simulink model "ThreePhase_Energy"  (R2024b)
settings: Solver=FixedStepAuto  StartTime=0.0  StopTime=Tsim  FixedStep=1e-5  RelTol=1e-3
values from neighbouring files (symbols this model uses):
  C = 2e-3    (= 0.002)    [PR_init_run.m]    (also in PowerClarke.m = [1 1 1;1 -1 0; 1 0 -1;])
  eng_ki = 1000    [PR_init_run.m]
  eng_kp = 20    [PR_init_run.m]
  Eref1 = 3*(0.5)*C*Vdc^2    (= 1920)    [PR_init_run.m]
  Eref2 = 0    [PR_init_run.m]
  Eref3 = 0    [PR_init_run.m]
  f = 50    [PR_init_run.m]
  Ki = 120    [PR_init_run.m]
  ki = 1000    [PR_init_run.m]
  Kp = 1    [PR_init_run.m]
  kp = 20    [PR_init_run.m]
  L = 1.3e-3    (= 0.0013)    [PR_init_run.m]
  max_i = 30    [PR_init_run.m]
  P = 10e3    (= 10000)    [PR_init_run.m]
  Ptrf = [1 1 1;1 -1 0; 1 0 -1;]    [PR_init_run.m]
  Q = 0    [PR_init_run.m]    (also in SOGI_bode.m = 3)
  Q1ref = -15e3    (= -15000)    [PR_init_run.m]
  R = 1e-2    (= 0.01)    [PR_init_run.m]
  Rcap = 50e-3    (= 0.05)    [PR_init_run.m]
  sogi_ki = 30    [PR_init_run.m]
  sogi_kp = 0.5    [PR_init_run.m]
  Tdist = 0.3    [PR_init_run.m]
  TQ = 0.08    [PR_init_run.m]
  Tstep = 0.06    [PR_init_run.m]
  Vdc = 800    [PR_init_run.m]
  Vpeak = V2*sqrt(2)    [PR_init_run.m]
  w = 2*pi*f    (= 314.159265359)    [PR_init_run.m]    (also in SOGI_bode.m)
  wc = 0.6283    [PR_init_run.m]
libraries: spsControlledVoltageSourceLib x9, simulink x4, spsControlledCurrentSourceLib x3, spsCurrentMeasurementLib x3, spsSeriesRLCBranchLib x3, spsVoltageMeasurementLib x3, spsAlphaBetaZerotodq0Lib x2, spsThreePhaseVIMeasurementLib x2, spsGroundLib x1, spsThreePhaseSeriesRLCBranchLib x1, sps_lib x1
settings Model: Creator=sproj  LastModifiedBy=sproj

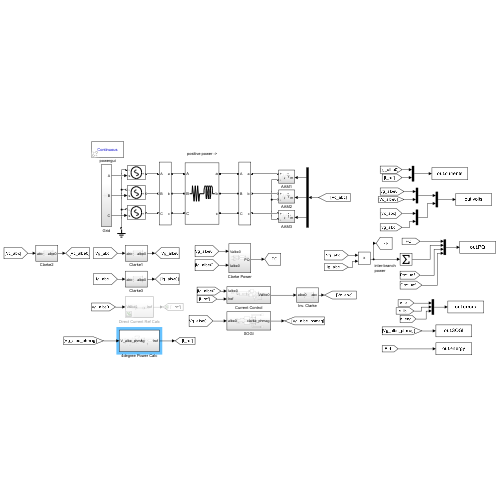
[thumbnail: Simulink's stored preview of the top-level diagram]
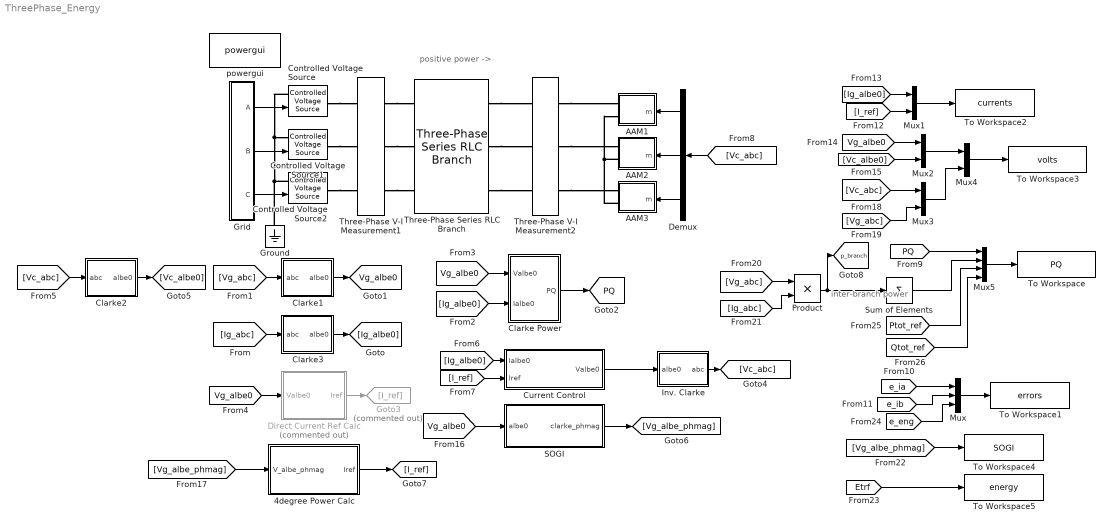
== system ThreePhase_Energy ==
  note: positive power ->
  note: inter-branch
      | power
  4degree Power Calc : Subsystem
  AAM1 : Subsystem
  AAM2 : Subsystem
  AAM3 : Subsystem
  Clarke Power : Subsystem
  Clarke1 : Subsystem
  Clarke2 : Subsystem
  Clarke3 : Subsystem
  Controlled Voltage Source : spsControlledVoltageSourceLib/Controlled Voltage Source  Initialize=on  Source_Type=AC  Amplitude=0  Phase=0  Frequency=0  Measurements=None
  Controlled Voltage Source1 : spsControlledVoltageSourceLib/Controlled Voltage Source  Initialize=on  Source_Type=AC  Amplitude=0  Phase=0  Frequency=0  Measurements=None
  Controlled Voltage Source2 : spsControlledVoltageSourceLib/Controlled Voltage Source  Initialize=on  Source_Type=AC  Amplitude=0  Phase=0  Frequency=0  Measurements=None
  Current Control : Subsystem
  Demux : Demux  Outputs=3
  Direct Current Ref Calc : Subsystem  Commented=on
  Goto3 : Goto  Commented=on  GotoTag=I_ref
  Grid : Subsystem
  Ground : spsGroundLib/Ground  LConnTagsString=a
  Inv. Clarke : Subsystem
  Mux : Mux  Inputs=3
  Mux{1..4} (4 alike) : Mux  Inputs=2
  Mux5 : Mux
  Product : Product
  SOGI : Subsystem
  Sum of Elements : Sum  Inputs=+
  Three-Phase Series RLC Branch : spsThreePhaseSeriesRLCBranchLib/Three-Phase Series RLC Branch  LConnTagsString=A|B|C  RConnTagsString=A|B|C  BranchType=RL  Resistance=R  Inductance=L  Capacitance=1e-6  Measurements=None
  Three-Phase V-I Measurement1 : spsThreePhaseVIMeasurementLib/Three-Phase V-I Measurement  VoltageMeasurement=phase-to-ground  SetLabelV=on  LabelV=Vg_abc  Vpu=off  VpuLL=off  CurrentMeasurement=yes  SetLabelI=on  LabelI=Ig_abc  Ipu=off  Pbase=100e6  Vbase=500e3  OutputType=Complex  PhasorSimulation=off  PSBequivalent=0
  Three-Phase V-I Measurement2 : spsThreePhaseVIMeasurementLib/Three-Phase V-I Measurement  VoltageMeasurement=phase-to-ground  SetLabelV=on  LabelV=Vc_abc  Vpu=off  VpuLL=off  CurrentMeasurement=yes  SetLabelI=on  LabelI=Ic_abc  Ipu=off  Pbase=100e6  Vbase=500e3  OutputType=Complex  PhasorSimulation=off  PSBequivalent=0
  To Workspace : ToWorkspace  VariableName=PQ  SaveFormat=Structure With Time  SampleTime=-1
  To Workspace1 : ToWorkspace  VariableName=errors  SaveFormat=Structure With Time  SampleTime=-1
  To Workspace2 : ToWorkspace  VariableName=currents  SaveFormat=Structure With Time  SampleTime=-1
  To Workspace3 : ToWorkspace  VariableName=volts  SaveFormat=Structure With Time  SampleTime=-1
  To Workspace4 : ToWorkspace  VariableName=SOGI  SaveFormat=Structure With Time  SampleTime=-1
  To Workspace5 : ToWorkspace  VariableName=energy  SaveFormat=Structure With Time  SampleTime=-1
  powergui : sps_lib/powergui  Priority=1  SimulationMode=Continuous  SampleTime=50e-6  frequency=60  Iterations=50  frequencyindice=0  Pbase=100e6  ErrMax=1e-4  UnitsV=kV  UnitsW=MW  buscounter=0  FunctionMessages=off  echomessages=off  EnableUseOfTLC=off  CurrentSourceSwitches=off  DisableSnubberDevices=off  DisableRonSwitches=off  DisableVfSwitches=off  DisplayEquations=off  AutomaticDiscreteSolvers=off  SolverType=Tustin/Backward Euler (TBE)  Interpol=off  ExternalGateDelay=off  methode=off  Ts=100  x0status=blocks  SPID=on  SwTol=0  HookPort=off  NonlinearTolerance=1e-4  nMaxIteration=100  ContinueOnMaxIteration=off  RestoreLinks=warning  ResistiveCurrentMeasurement=off  Frange=[0:2:500]  Ylog=off  Xlog=on  ShowGrid=off  save=off  variable=ZData  structure=0  ZoomFFT=off  StartTime=0.0  cycles=1  DisplayStyle=1  fundamental=60  FreqAxis=off  MaxFrequency=1000  frequencyindicesteady=1  RmsSteady=1  display=off
  tag scope: PQ=global, Vg_albe0=global, p_branch=global
  wires:
  Grid/2(B) -> Controlled Voltage Source1/1
  Grid/1(A) -> Controlled Voltage Source/1
  Grid/3(C) -> Controlled Voltage Source2/1
  [Ig_abc] -> Clarke3/1(abc)
  Clarke3/1(albe0) -> [Ig_albe0]
  [Vg_abc] -> Clarke1/1(abc)
  Clarke1/1(albe0) -> [Vg_albe0]
  [Ig_albe0] -> Clarke Power/2(Ialbe0)
  [Vg_albe0] -> Clarke Power/1(Valbe0)
  [Vg_albe0] -> Direct Current Ref Calc/1(Valbe0)
  Clarke Power/1(PQ) -> [PQ]
  [Ig_albe0] -> Current Control/1(Ialbe0)
  Direct Current Ref Calc/1(Iref) -> Goto3/1
  [I_ref] -> Current Control/2(Iref)
  Inv. Clarke/1(abc) -> [Vc_abc]
  [Vc_abc] -> Demux/1
  [e_ia] -> Mux/1
  [e_ib] -> Mux/2
  Mux/1 -> To Workspace1/1
  [Ig_albe0] -> Mux1/1
  [I_ref] -> Mux1/2
  Mux1/1 -> To Workspace2/1
  Current Control/1(Valbe0) -> Inv. Clarke/1(albe0)
  Demux/2 -> AAM2/1(m)
  Demux/1 -> AAM1/1(m)
  Demux/3 -> AAM3/1(m)
  [Vg_albe0] -> Mux2/1
  Clarke2/1(albe0) -> [Vc_albe0]
  [Vc_abc] -> Clarke2/1(abc)
  [Vc_albe0] -> Mux2/2
  [Vg_albe0] -> SOGI/1(albe0)
  SOGI/1(clarke_phmag) -> [Vg_albe_phmag]
  [Vg_albe_phmag] -> 4degree Power Calc/1(V_albe_phmag)
  [Vc_abc] -> Mux3/1
  [Vg_abc] -> Mux3/2
  Mux2/1 -> Mux4/1
  Mux3/1 -> Mux4/2
  Mux4/1 -> To Workspace3/1
  [Vg_abc] -> Product/1
  [Ig_abc] -> Product/2
  Product/1 -> Sum of Elements/1, [p_branch]
  [PQ] -> Mux5/1
  Sum of Elements/1 -> Mux5/2
  Mux5/1 -> To Workspace/1
  4degree Power Calc/1(Iref) -> [I_ref]
  [Vg_albe_phmag] -> To Workspace4/1
  [Etrf] -> To Workspace5/1
  [e_eng] -> Mux/3
  [Ptot_ref] -> Mux5/3
  [Qtot_ref] -> Mux5/4
  connections:
  Controlled Voltage Source1/LConn1 -- Controlled Voltage Source2/LConn1 -- Ground/LConn1 -- Controlled Voltage Source/LConn1
  Three-Phase Series RLC Branch/RConn1 -- Three-Phase V-I Measurement2/LConn1
  Three-Phase Series RLC Branch/RConn2 -- Three-Phase V-I Measurement2/LConn2
  Three-Phase Series RLC Branch/RConn3 -- Three-Phase V-I Measurement2/LConn3
  Three-Phase V-I Measurement2/RConn3 -- AAM3/RConn1
  Three-Phase V-I Measurement2/RConn2 -- AAM2/RConn1
  Three-Phase V-I Measurement2/RConn1 -- AAM1/RConn1
  Controlled Voltage Source/RConn1 -- Three-Phase V-I Measurement1/LConn1
  Controlled Voltage Source1/RConn1 -- Three-Phase V-I Measurement1/LConn2
  Controlled Voltage Source2/RConn1 -- Three-Phase V-I Measurement1/LConn3
  Three-Phase V-I Measurement1/RConn1 -- Three-Phase Series RLC Branch/LConn1
  Three-Phase V-I Measurement1/RConn2 -- Three-Phase Series RLC Branch/LConn2
  Three-Phase V-I Measurement1/RConn3 -- Three-Phase Series RLC Branch/LConn3
  AAM2/RConn2 -- AAM1/RConn2 -- AAM3/RConn2

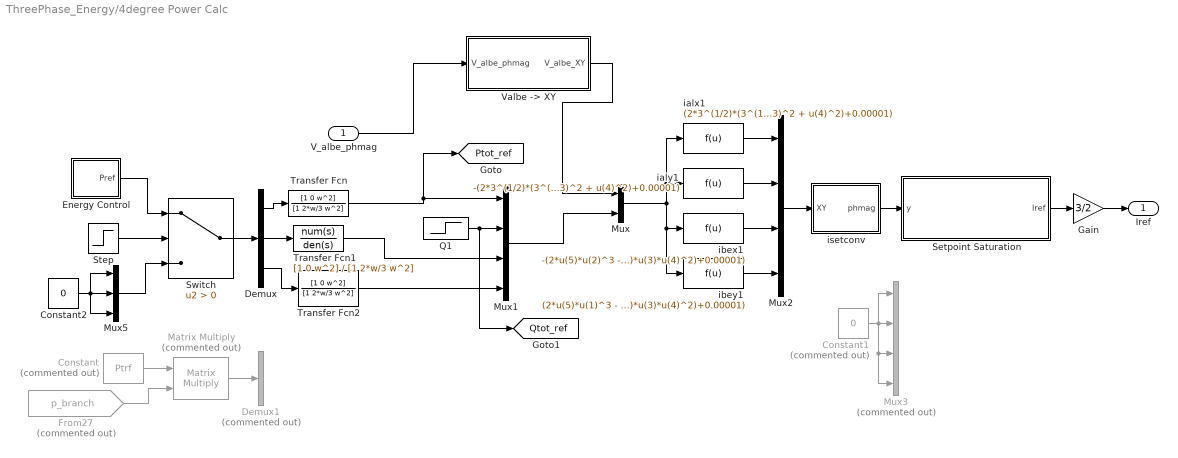
== system ThreePhase_Energy/4degree Power Calc ==
  V_albe_phmag : Inport
  Constant : Constant  Commented=on  Value=Ptrf
  Constant1 : Constant  Commented=on  Value=0
  Constant2 : Constant  Value=0
  Demux : Demux  Outputs=3
  Demux1 : Demux  Commented=on  Outputs=3
  Energy Control : Subsystem
  From27 : From  Commented=on  GotoTag=p_branch  TagVisibility=global
  Gain : Gain  Gain=3/2
  Matrix Multiply : Product  Commented=on  Multiplication=Matrix(*)
  Mux : Mux  Inputs=2
  Mux1 : Mux
  Mux2 : Mux
  Mux3 : Mux  Commented=on
  Mux5 : Mux  Inputs=3
  Q1 : Step  Time=TQ  After=Q1ref  SampleTime=0
  Setpoint Saturation : Subsystem
  Step : Step  Time=Tstep  SampleTime=0
  Switch : Switch  Criteria=u2 > Threshold  SaturateOnIntegerOverflow=off  InputSameDT=off
  Transfer Fcn : TransferFcn  Numerator=[1 0 w^2]  Denominator=[1 2*w/3 w^2]
  Transfer Fcn1 : TransferFcn  Numerator=[1 0 w^2]  Denominator=[1 2*w/3 w^2]
  Transfer Fcn2 : TransferFcn  Numerator=[1 0 w^2]  Denominator=[1 2*w/3 w^2]
  "Valbe -> XY" : Subsystem
  ialx1 : Fcn  Expr=(2*3^(1/2)*(3^(1/2)*u(5)*u(4)^3 + 3^(1/2)*u(7)*u(4)^3 + 3^(1/2)*u(8)*u(4)^3 - 6*u(7)*u(2)*u(3)^2 - 6*u(7)*u(2)*u(4)^2 + 6*u(8)*u(2)*u(3)^2 + 6*u(8)*u(2)*u(4)^2 + 3^(1/2)*u(5)*u(1)^2*u(4) + 3^(1/2)*u(5)*u(2)^2*u(4) + 3^(1/2)*u(7)*u(1)^2*u(4) - 3^(1/2)*u(7)*u(2)^2*u(4) + 3^(1/2)*u(8)*u(1)^2*u(4) - 3^(1/2)*u(8)*u(2)^2*u(4) + 3^(1/2)*u(5)*u(3)^2*u(4) + 3^(1/2)*u(7)*u(3)^2*u(4) + 3^(1/2)*u(8)*u(3)^2*u(4) - 2*3^(1/2)*u(6)*u(2)^2*u(3) - 2*3^(1/2)*u(7)*u(1)*u(2)*u(3) - 2*3^(1/2)*u(8)*u(1)*u(2)*u(3) + 2*3^(1/2)*u(6)*u(1)*u(2)*u(4)))/(9*(u(1)*u(4) - u(2)*u(3))*(u(1)^2 + u(2)^2 + u(3)^2 + u(4)^2)+0.00001)
  ialy1 : Fcn  Expr=-(2*3^(1/2)*(3^(1/2)*u(5)*u(3)^3 + 3^(1/2)*u(7)*u(3)^3 + 3^(1/2)*u(8)*u(3)^3 - 6*u(7)*u(1)*u(3)^2 - 6*u(7)*u(1)*u(4)^2 + 6*u(8)*u(1)*u(3)^2 + 6*u(8)*u(1)*u(4)^2 + 3^(1/2)*u(5)*u(1)^2*u(3) + 3^(1/2)*u(5)*u(2)^2*u(3) - 3^(1/2)*u(7)*u(1)^2*u(3) + 3^(1/2)*u(7)*u(2)^2*u(3) - 3^(1/2)*u(8)*u(1)^2*u(3) + 3^(1/2)*u(8)*u(2)^2*u(3) + 3^(1/2)*u(5)*u(3)*u(4)^2 + 3^(1/2)*u(7)*u(3)*u(4)^2 + 3^(1/2)*u(8)*u(3)*u(4)^2 + 2*3^(1/2)*u(6)*u(1)^2*u(4) - 2*3^(1/2)*u(7)*u(1)*u(2)*u(4) - 2*3^(1/2)*u(8)*u(1)*u(2)*u(4) - 2*3^(1/2)*u(6)*u(1)*u(2)*u(3)))/(9*(u(1)*u(4) - u(2)*u(3))*(u(1)^2 + u(2)^2 + u(3)^2 + u(4)^2)+0.00001)
  ibex1 : Fcn  Expr=-(2*u(5)*u(2)^3 - 2*u(7)*u(2)^3 - 2*u(8)*u(2)^3 + 2*u(5)*u(1)^2*u(2) - 2*u(7)*u(1)^2*u(2) - 2*u(8)*u(1)^2*u(2) + 2*u(5)*u(2)*u(3)^2 + 2*u(5)*u(2)*u(4)^2 - 2*u(7)*u(2)*u(3)^2 + 2*u(7)*u(2)*u(4)^2 - 2*u(8)*u(2)*u(3)^2 + 2*u(8)*u(2)*u(4)^2 - 4*u(6)*u(1)*u(4)^2 + 4*u(7)*u(1)*u(3)*u(4) + 4*u(8)*u(1)*u(3)*u(4) + 4*u(6)*u(2)*u(3)*u(4) - 4*3^(1/2)*u(7)*u(1)^2*u(4) - 4*3^(1/2)*u(7)*u(2)^2*u(4) + 4*3^(1/2)*u(8)*u(1)^2*u(4) + 4*3^(1/2)*u(8)*u(2)^2*u(4))/(3*(u(1)^3*u(4) - u(1)^2*u(2)*u(3) + u(1)*u(2)^2*u(4) + u(1)*u(3)^2*u(4) + u(1)*u(4)^3 - u(2)^3*u(3) - u(2)*u(3)^3 - u(2)*u(3)*u(4)^2)+0.00001)
  ibey1 : Fcn  Expr=(2*u(5)*u(1)^3 - 2*u(7)*u(1)^3 - 2*u(8)*u(1)^3 + 2*u(5)*u(1)*u(2)^2 - 2*u(7)*u(1)*u(2)^2 - 2*u(8)*u(1)*u(2)^2 + 2*u(5)*u(1)*u(3)^2 + 2*u(5)*u(1)*u(4)^2 + 2*u(7)*u(1)*u(3)^2 - 2*u(7)*u(1)*u(4)^2 + 2*u(8)*u(1)*u(3)^2 - 2*u(8)*u(1)*u(4)^2 + 4*u(6)*u(2)*u(3)^2 + 4*u(7)*u(2)*u(3)*u(4) + 4*u(8)*u(2)*u(3)*u(4) - 4*u(6)*u(1)*u(3)*u(4) - 4*3^(1/2)*u(7)*u(1)^2*u(3) - 4*3^(1/2)*u(7)*u(2)^2*u(3) + 4*3^(1/2)*u(8)*u(1)^2*u(3) + 4*3^(1/2)*u(8)*u(2)^2*u(3))/(3*(u(1)^3*u(4) - u(1)^2*u(2)*u(3) + u(1)*u(2)^2*u(4) + u(1)*u(3)^2*u(4) + u(1)*u(4)^3 - u(2)^3*u(3) - u(2)*u(3)^3 - u(2)*u(3)*u(4)^2)+0.00001)
  isetconv : Subsystem
  Iref : Outport
  tag scope: Ptot_ref=global, Qtot_ref=global
  wires:
  V_albe_phmag/1 -> "Valbe -> XY"/1(V_albe_phmag)
  Q1/1 -> [Qtot_ref], Mux1/2
  "Valbe -> XY"/1(V_albe_XY) -> Mux/1
  Mux1/1 -> Mux/2
  Mux/1 -> ibey1/1, ibex1/1, ialy1/1, ialx1/1
  Mux2/1 -> isetconv/1(XY)
  Constant1/1 -> Mux3/1, Mux3/4, Mux3/3, Mux3/2
  ialx1/1 -> Mux2/1
  ialy1/1 -> Mux2/2
  ibex1/1 -> Mux2/3
  ibey1/1 -> Mux2/4
  isetconv/1(phmag) -> Setpoint Saturation/1(y)
  Setpoint Saturation/1(Iref) -> Gain/1
  Gain/1 -> Iref/1
  Switch/1 -> Demux/1
  Step/1 -> Switch/2
  Constant2/1 -> Mux5/3, Mux5/1, Mux5/2
  Energy Control/1(Pref) -> Switch/1
  Mux5/1 -> Switch/3
  Demux/1 -> Transfer Fcn/1
  Demux/3 -> Transfer Fcn2/1
  Constant/1 -> Matrix Multiply/1
  From27/1 -> Matrix Multiply/2
  Matrix Multiply/1 -> Demux1/1
  Demux/2 -> Transfer Fcn1/1
  Transfer Fcn/1 -> [Ptot_ref], Mux1/1
  Transfer Fcn1/1 -> Mux1/3
  Transfer Fcn2/1 -> Mux1/4

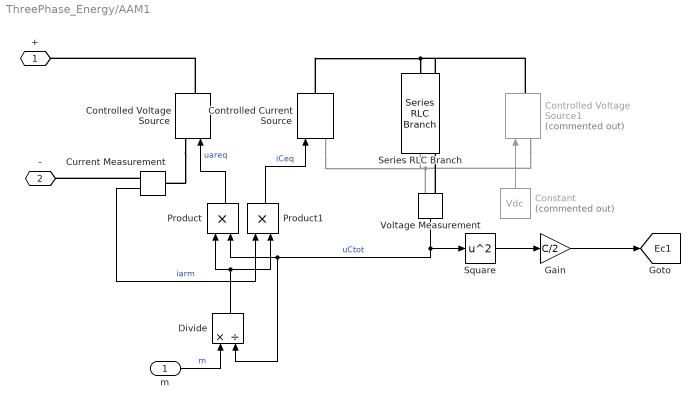
== system ThreePhase_Energy/AAM1 ==
  m : Inport
  Constant : Constant  Commented=on  Value=Vdc
  Controlled Current Source : spsControlledCurrentSourceLib/Controlled Current Source  Initialize=on  Source_Type=AC  Amplitude=0  Phase=0  Frequency=0  Measurements=None
  Controlled Voltage Source : spsControlledVoltageSourceLib/Controlled Voltage Source  Initialize=on  Source_Type=AC  Amplitude=0  Phase=0  Frequency=0  Measurements=None
  Controlled Voltage Source1 : spsControlledVoltageSourceLib/Controlled Voltage Source  Commented=on  Initialize=on  Source_Type=DC  Amplitude=400  Phase=0  Frequency=0  Measurements=None
  Current Measurement : spsCurrentMeasurementLib/Current Measurement  PhasorSimulation=off  OutputType=Complex  PSBequivalent=0
  Divide : Product  Inputs=*/
  Gain : Gain  Gain=C/2
  Product : Product
  Product1 : Product
  Series RLC Branch : spsSeriesRLCBranchLib/Series RLC Branch  LConnTagsString=__new0  RConnTagsString=__new0  BranchType=RC  Resistance=Rcap  Inductance=1e-3  SetiL0=off  InitialCurrent=0  Capacitance=C  Setx0=on  InitialVoltage=Vdc  Measurements=None
  Square : Math  Operator=square
  Voltage Measurement : spsVoltageMeasurementLib/Voltage Measurement  PhasorSimulation=off  OutputType=Complex  PSBequivalent=0
  + : PMIOPort  Side=Right
  - : PMIOPort  Port=2  Side=Right
  tag scope: Ec1=global
  wires:
  Product/1 -> Controlled Voltage Source/1  "uareq"
  Voltage Measurement/1 -> Square/1, Divide/2, Product/2  "uCtot"
  Product1/1 -> Controlled Current Source/1  "iCeq"
  Current Measurement/1 -> Product1/1  "iarm"
  Constant/1 -> Controlled Voltage Source1/1
  m/1 -> Divide/1  "m"
  Divide/1 -> Product/1, Product1/2
  Square/1 -> Gain/1
  Gain/1 -> [Ec1]
  connections:
  Controlled Voltage Source1/LConn1 -- Voltage Measurement/LConn2 -- Controlled Current Source/LConn1 -- Series RLC Branch/RConn1
  Controlled Voltage Source/RConn1 -- +/RConn1
  Controlled Current Source/RConn1 -- Series RLC Branch/LConn1 -- Voltage Measurement/LConn1 -- Controlled Voltage Source1/RConn1
  Controlled Voltage Source/LConn1 -- Current Measurement/LConn1
  Current Measurement/RConn1 -- -/RConn1

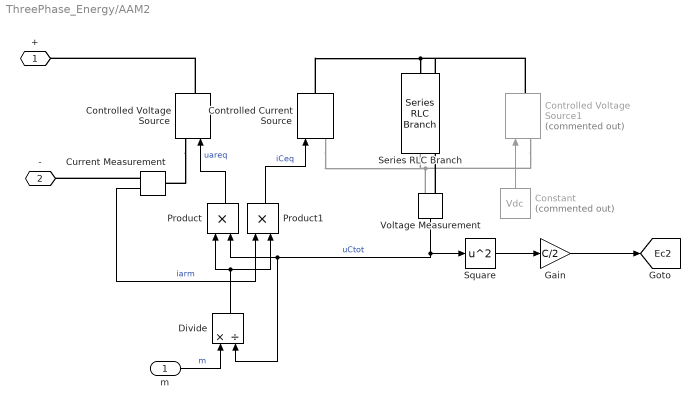
== system ThreePhase_Energy/AAM2 ==
  m : Inport
  Constant : Constant  Commented=on  Value=Vdc
  Controlled Current Source : spsControlledCurrentSourceLib/Controlled Current Source  Initialize=on  Source_Type=AC  Amplitude=0  Phase=0  Frequency=0  Measurements=None
  Controlled Voltage Source : spsControlledVoltageSourceLib/Controlled Voltage Source  Initialize=on  Source_Type=AC  Amplitude=0  Phase=0  Frequency=0  Measurements=None
  Controlled Voltage Source1 : spsControlledVoltageSourceLib/Controlled Voltage Source  Commented=on  Initialize=on  Source_Type=DC  Amplitude=400  Phase=0  Frequency=0  Measurements=None
  Current Measurement : spsCurrentMeasurementLib/Current Measurement  PhasorSimulation=off  OutputType=Complex  PSBequivalent=0
  Divide : Product  Inputs=*/
  Gain : Gain  Gain=C/2
  Product : Product
  Product1 : Product
  Series RLC Branch : spsSeriesRLCBranchLib/Series RLC Branch  LConnTagsString=__new0  RConnTagsString=__new0  BranchType=RC  Resistance=Rcap  Inductance=1e-3  SetiL0=off  InitialCurrent=0  Capacitance=C  Setx0=on  InitialVoltage=Vdc  Measurements=None
  Square : Math  Operator=square
  Voltage Measurement : spsVoltageMeasurementLib/Voltage Measurement  PhasorSimulation=off  OutputType=Complex  PSBequivalent=0
  + : PMIOPort  Side=Right
  - : PMIOPort  Port=2  Side=Right
  tag scope: Ec2=global
  wires:
  Product/1 -> Controlled Voltage Source/1  "uareq"
  Voltage Measurement/1 -> Square/1, Divide/2, Product/2  "uCtot"
  Product1/1 -> Controlled Current Source/1  "iCeq"
  Current Measurement/1 -> Product1/1  "iarm"
  Constant/1 -> Controlled Voltage Source1/1
  m/1 -> Divide/1  "m"
  Divide/1 -> Product/1, Product1/2
  Square/1 -> Gain/1
  Gain/1 -> [Ec2]
  connections:
  Controlled Voltage Source1/LConn1 -- Voltage Measurement/LConn2 -- Controlled Current Source/LConn1 -- Series RLC Branch/RConn1
  Controlled Voltage Source/RConn1 -- +/RConn1
  Controlled Current Source/RConn1 -- Series RLC Branch/LConn1 -- Voltage Measurement/LConn1 -- Controlled Voltage Source1/RConn1
  Controlled Voltage Source/LConn1 -- Current Measurement/LConn1
  Current Measurement/RConn1 -- -/RConn1

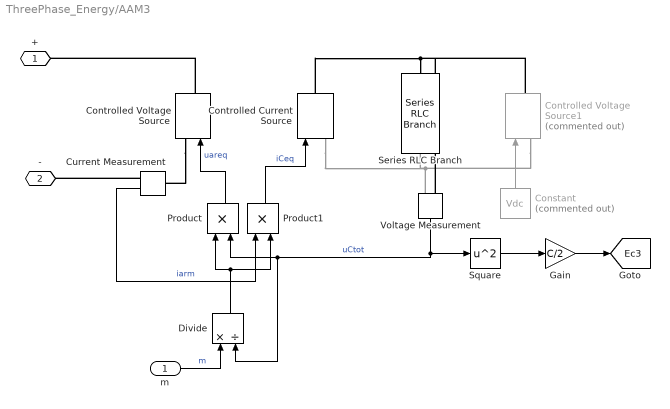
== system ThreePhase_Energy/AAM3 ==
  m : Inport
  Constant : Constant  Commented=on  Value=Vdc
  Controlled Current Source : spsControlledCurrentSourceLib/Controlled Current Source  Initialize=on  Source_Type=AC  Amplitude=0  Phase=0  Frequency=0  Measurements=None
  Controlled Voltage Source : spsControlledVoltageSourceLib/Controlled Voltage Source  Initialize=on  Source_Type=AC  Amplitude=0  Phase=0  Frequency=0  Measurements=None
  Controlled Voltage Source1 : spsControlledVoltageSourceLib/Controlled Voltage Source  Commented=on  Initialize=on  Source_Type=DC  Amplitude=400  Phase=0  Frequency=0  Measurements=None
  Current Measurement : spsCurrentMeasurementLib/Current Measurement  PhasorSimulation=off  OutputType=Complex  PSBequivalent=0
  Divide : Product  Inputs=*/
  Gain : Gain  Gain=C/2
  Product : Product
  Product1 : Product
  Series RLC Branch : spsSeriesRLCBranchLib/Series RLC Branch  LConnTagsString=__new0  RConnTagsString=__new0  BranchType=RC  Resistance=Rcap  Inductance=1e-3  SetiL0=off  InitialCurrent=0  Capacitance=C  Setx0=on  InitialVoltage=Vdc  Measurements=None
  Square : Math  Operator=square
  Voltage Measurement : spsVoltageMeasurementLib/Voltage Measurement  PhasorSimulation=off  OutputType=Complex  PSBequivalent=0
  + : PMIOPort  Side=Right
  - : PMIOPort  Port=2  Side=Right
  tag scope: Ec3=global
  wires:
  Product/1 -> Controlled Voltage Source/1  "uareq"
  Voltage Measurement/1 -> Square/1, Divide/2, Product/2  "uCtot"
  Product1/1 -> Controlled Current Source/1  "iCeq"
  Current Measurement/1 -> Product1/1  "iarm"
  Constant/1 -> Controlled Voltage Source1/1
  m/1 -> Divide/1  "m"
  Divide/1 -> Product/1, Product1/2
  Square/1 -> Gain/1
  Gain/1 -> [Ec3]
  connections:
  Controlled Voltage Source1/LConn1 -- Voltage Measurement/LConn2 -- Controlled Current Source/LConn1 -- Series RLC Branch/RConn1
  Controlled Voltage Source/RConn1 -- +/RConn1
  Controlled Current Source/RConn1 -- Voltage Measurement/LConn1 -- Controlled Voltage Source1/RConn1 -- Series RLC Branch/LConn1
  Controlled Voltage Source/LConn1 -- Current Measurement/LConn1
  Current Measurement/RConn1 -- -/RConn1

== system ThreePhase_Energy/Clarke Power ==
  Valbe0 : Inport
  Ialbe0 : Inport  Port=2
  Demux : Demux  Outputs=3
  Demux1 : Demux  Outputs=3
  Fcn : Fcn  Expr=u(1)*u(3) + u(2)*u(4)
  Fcn1 : Fcn  Expr=-u(1)*u(4) + u(2)*u(3)
  Mux : Mux
  Mux1 : Mux  Inputs=2
  Terminator : Terminator
  Terminator1 : Terminator
  PQ : Outport
  wires:
  Demux/1 -> Mux/1  "val"
  Mux/1 -> Fcn/1, Fcn1/1
  Demux1/3 -> Terminator1/1
  Valbe0/1 -> Demux/1
  Demux/3 -> Terminator/1
  Demux/2 -> Mux/2  "vbe"
  Demux1/2 -> Mux/4  "ibe"
  Demux1/1 -> Mux/3  "ial"
  Ialbe0/1 -> Demux1/1
  Fcn1/1 -> Mux1/2  "Q"
  Fcn/1 -> Mux1/1  "P"
  Mux1/1 -> PQ/1

== system ThreePhase_Energy/Clarke1 ==
  abc : Inport
  Fcn : Fcn  Expr=2*u(1) - u(2) - u(3)
  Fcn1 : Fcn  Expr=sqrt(3)*u(2) - sqrt(3)*u(3)
  Fcn2 : Fcn  Expr=u(1) + u(2) + u(3)
  Gain : Gain  Gain=1/3
  Mux : Mux  Inputs=3
  albe0 : Outport
  wires:
  Fcn/1 -> Mux/1
  Fcn2/1 -> Mux/3
  Fcn1/1 -> Mux/2
  abc/1 -> Gain/1
  Gain/1 -> Fcn1/1, Fcn/1, Fcn2/1
  Mux/1 -> albe0/1

== system ThreePhase_Energy/Clarke2 ==
  abc : Inport
  Fcn : Fcn  Expr=2*u(1) - u(2) - u(3)
  Fcn1 : Fcn  Expr=sqrt(3)*u(2) - sqrt(3)*u(3)
  Fcn2 : Fcn  Expr=u(1) + u(2) + u(3)
  Gain : Gain  Gain=1/3
  Mux : Mux  Inputs=3
  albe0 : Outport
  wires:
  Mux/1 -> albe0/1
  Gain/1 -> Fcn2/1, Fcn/1, Fcn1/1
  abc/1 -> Gain/1
  Fcn1/1 -> Mux/2
  Fcn2/1 -> Mux/3
  Fcn/1 -> Mux/1

== system ThreePhase_Energy/Clarke3 ==
  abc : Inport
  Fcn : Fcn  Expr=2*u(1) - u(2) - u(3)
  Fcn1 : Fcn  Expr=sqrt(3)*u(2) - sqrt(3)*u(3)
  Fcn2 : Fcn  Expr=u(1) + u(2) + u(3)
  Gain : Gain  Gain=1/3
  Mux : Mux  Inputs=3
  albe0 : Outport
  wires:
  Mux/1 -> albe0/1
  Gain/1 -> Fcn2/1, Fcn/1, Fcn1/1
  abc/1 -> Gain/1
  Fcn1/1 -> Mux/2
  Fcn2/1 -> Mux/3
  Fcn/1 -> Mux/1

== system ThreePhase_Energy/Current Control ==
  Ialbe0 : Inport
  Iref : Inport  Port=2
  Constant : Constant  Value=0
  Demux : Demux  Outputs=3
  Demux1 : Demux  Outputs=2
  Mux : Mux  Inputs=3
  PR : Subsystem
  PR1 : Subsystem
  Sum : Sum  Inputs=|++
  Terminator : Terminator
  Valbe0 : Outport
  wires:
  Demux/1 -> PR/2(meas)
  Iref/1 -> Demux1/1
  Demux1/2 -> PR1/1(ref)
  Demux/2 -> PR1/2(meas)
  PR/1(out) -> Mux/1
  Demux/3 -> Terminator/1
  PR1/1(out) -> Mux/2
  Ialbe0/1 -> Demux/1
  Constant/1 -> Mux/3
  Sum/1 -> Valbe0/1
  [Vg_albe0] -> Sum/2
  Mux/1 -> Sum/1
  Demux1/1 -> PR/1(ref)

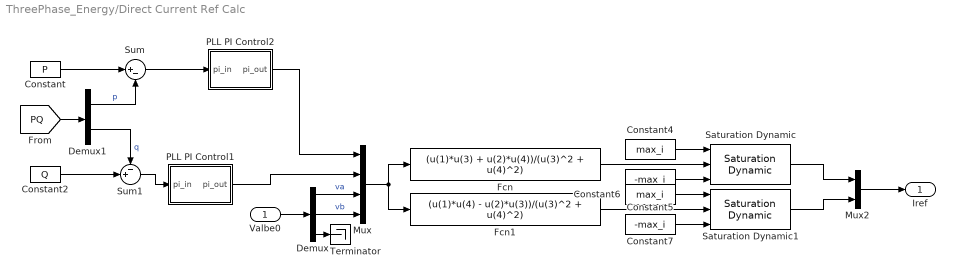
== system ThreePhase_Energy/Direct Current Ref Calc ==
  Valbe0 : Inport
  Constant : Constant  Value=P
  Constant2 : Constant  Value=Q
  Constant4 : Constant  Value=max_i
  Constant5 : Constant  Value=-max_i
  Constant6 : Constant  Value=max_i
  Constant7 : Constant  Value=-max_i
  Demux : Demux  Outputs=3
  Demux1 : Demux  Outputs=2
  Fcn : Fcn  Expr=(u(1)*u(3) + u(2)*u(4))/(u(3)^2 + u(4)^2)
  Fcn1 : Fcn  Expr=(u(1)*u(4) - u(2)*u(3))/(u(3)^2 + u(4)^2)
  Mux : Mux
  Mux2 : Mux  Inputs=2
  PLL PI Control1 : Subsystem
  PLL PI Control2 : Subsystem
  Saturation Dynamic : simulink/Discontinuities/Saturation Dynamic  OutMin=[]  OutMax=[]  OutDataTypeStr=Inherit: Same as second input  OutDataType=fixdt(1, 16)  OutScaling=2^-10  DoSatur=off
  Saturation Dynamic1 : simulink/Discontinuities/Saturation Dynamic  OutMin=[]  OutMax=[]  OutDataTypeStr=Inherit: Same as second input  OutDataType=fixdt(1, 16)  OutScaling=2^-10  DoSatur=off
  Sum : Sum  Inputs=|+-
  Sum1 : Sum  Inputs=-+|
  Terminator : Terminator
  Iref : Outport
  wires:
  Demux/3 -> Terminator/1
  Valbe0/1 -> Demux/1
  Demux/1 -> Mux/3  "va"
  Demux/2 -> Mux/4  "vb"
  Mux/1 -> Fcn1/1, Fcn/1
  [PQ] -> Demux1/1
  Constant/1 -> Sum/1
  Demux1/1 -> Sum/2  "p"
  Sum/1 -> PLL PI Control2/1(pi_in)
  PLL PI Control2/1(pi_out) -> Mux/1
  Constant2/1 -> Sum1/2
  Demux1/2 -> Sum1/1  "q"
  Sum1/1 -> PLL PI Control1/1(pi_in)
  PLL PI Control1/1(pi_out) -> Mux/2
  Saturation Dynamic/1 -> Mux2/1
  Fcn/1 -> Saturation Dynamic/2
  Fcn1/1 -> Saturation Dynamic1/2
  Constant5/1 -> Saturation Dynamic/3
  Constant6/1 -> Saturation Dynamic1/1
  Mux2/1 -> Iref/1
  Constant4/1 -> Saturation Dynamic/1
  Saturation Dynamic1/1 -> Mux2/2
  Constant7/1 -> Saturation Dynamic1/3

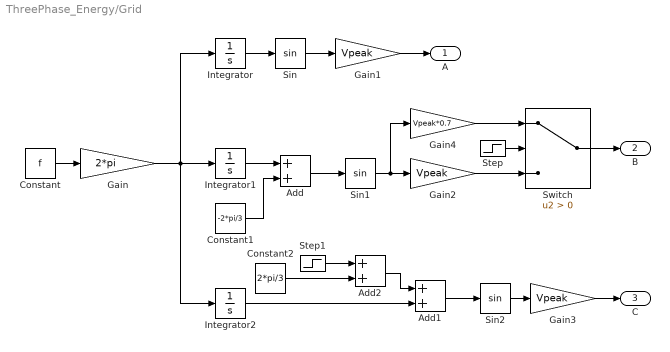
== system ThreePhase_Energy/Grid ==
  Add : Sum
  Add1 : Sum
  Add2 : Sum
  Constant : Constant  Value=f
  Constant1 : Constant  Value=-2*pi/3
  Constant2 : Constant  Value=2*pi/3
  Gain : Gain  Gain=2*pi
  Gain1 : Gain  Gain=Vpeak
  Gain2 : Gain  Gain=Vpeak
  Gain3 : Gain  Gain=Vpeak
  Gain4 : Gain  Gain=Vpeak*0.7
  Integrator : Integrator
  Integrator1 : Integrator
  Integrator2 : Integrator
  Sin : Trigonometry
  Sin1 : Trigonometry
  Sin2 : Trigonometry
  Step : Step  Time=Tdist  SampleTime=0
  Step1 : Step  Time=Tdist  After=pi/6  SampleTime=0
  Switch : Switch  Criteria=u2 > Threshold  SaturateOnIntegerOverflow=off  InputSameDT=off
  A : Outport
  B : Outport  Port=2
  C : Outport  Port=3
  wires:
  Constant1/1 -> Add/2
  Add1/1 -> Sin2/1
  Integrator1/1 -> Add/1
  Constant/1 -> Gain/1
  Integrator/1 -> Sin/1
  Gain/1 -> Integrator2/1, Integrator/1, Integrator1/1
  Add/1 -> Sin1/1
  Sin1/1 -> Gain4/1, Gain2/1
  Integrator2/1 -> Add1/2
  Step/1 -> Switch/2
  Gain2/1 -> Switch/3
  Gain4/1 -> Switch/1
  Switch/1 -> B/1
  Step1/1 -> Add2/1
  Constant2/1 -> Add2/2
  Add2/1 -> Add1/1
  Sin/1 -> Gain1/1
  Sin2/1 -> Gain3/1
  Gain1/1 -> A/1
  Gain3/1 -> C/1

== system ThreePhase_Energy/Inv. Clarke ==
  albe0 : Inport
  Fcn : Fcn  Expr="2*u(1) +  2*u(3)"
  Fcn1 : Fcn  Expr=-u(1) + sqrt(3)*u(2) + 2*u(3)
  Fcn2 : Fcn  Expr=-u(1) - sqrt(3)*u(2) + 2*u(3)
  Gain : Gain  Gain=1/2
  Mux : Mux  Inputs=3
  abc : Outport
  wires:
  Fcn/1 -> Mux/1
  Fcn2/1 -> Mux/3
  Fcn1/1 -> Mux/2
  albe0/1 -> Gain/1
  Gain/1 -> Fcn1/1, Fcn/1, Fcn2/1
  Mux/1 -> abc/1

== system ThreePhase_Energy/SOGI ==
  albe0 : Inport
  Demux1 : Demux  Outputs=3
  Mux3 : Mux
  SOGI PLL : Subsystem
  SOGI PLL1 : Subsystem
  Scope : Scope  Commented=on  NumInputPorts=2
  Scope1 : Scope  Commented=on  NumInputPorts=2
  Terminator : Terminator
  clarke_phmag : Outport
  wires:
  Demux1/1 -> SOGI PLL/1(in)  "alpha"
  SOGI PLL/1(theta) -> Scope/1, Mux3/1
  SOGI PLL/2(mag) -> Scope1/1, Mux3/2  "alpha"
  SOGI PLL1/1(theta) -> Scope/2, Mux3/3
  SOGI PLL1/2(mag) -> Scope1/2, Mux3/4  "beta"
  Demux1/2 -> SOGI PLL1/1(in)  "beta"
  albe0/1 -> Demux1/1
  Demux1/3 -> Terminator/1
  Mux3/1 -> clarke_phmag/1

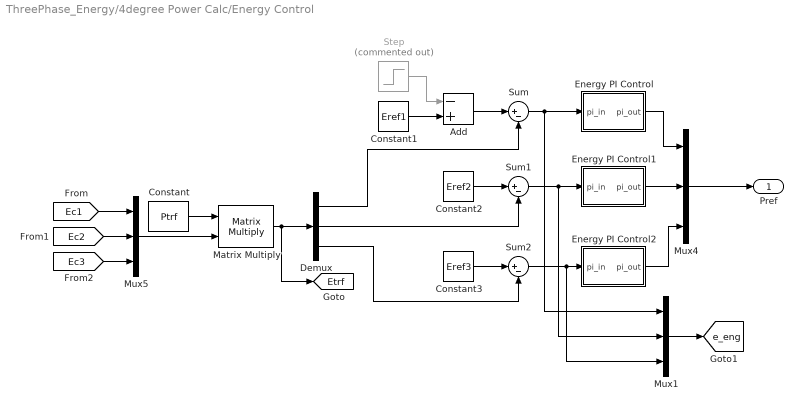
== system ThreePhase_Energy/4degree Power Calc/Energy Control ==
  Add : Sum  Inputs=-+
  Constant : Constant  Value=Ptrf
  Constant1 : Constant  Value=Eref1
  Constant2 : Constant  Value=Eref2
  Constant3 : Constant  Value=Eref3
  Demux : Demux  Outputs=3
  Energy PI Control : Subsystem
  Energy PI Control1 : Subsystem
  Energy PI Control2 : Subsystem
  Matrix Multiply : Product  Multiplication=Matrix(*)
  Mux1 : Mux  Inputs=3
  Mux4 : Mux  Inputs=3
  Mux5 : Mux  Inputs=3
  Step : Step  Commented=on  Time=Tdist  After=Eref1*0.15  SampleTime=0
  Sum : Sum  Inputs=|+-
  Sum1 : Sum  Inputs=|+-
  Sum2 : Sum  Inputs=|+-
  Pref : Outport
  tag scope: Etrf=global, e_eng=global
  wires:
  [Ec2] -> Mux5/2
  Constant3/1 -> Sum2/1
  [Ec1] -> Mux5/1
  Mux5/1 -> Matrix Multiply/2
  Matrix Multiply/1 -> [Etrf], Demux/1
  Sum1/1 -> Mux1/2, Energy PI Control1/1(pi_in)
  Sum/1 -> Mux1/1, Energy PI Control/1(pi_in)
  Constant2/1 -> Sum1/1
  Energy PI Control2/1(pi_out) -> Mux4/3
  Sum2/1 -> Mux1/3, Energy PI Control2/1(pi_in)
  Demux/3 -> Sum2/2
  [Ec3] -> Mux5/3
  Mux4/1 -> Pref/1
  Energy PI Control1/1(pi_out) -> Mux4/2
  Constant/1 -> Matrix Multiply/1
  Demux/1 -> Sum/2
  Demux/2 -> Sum1/2
  Mux1/1 -> [e_eng]
  Step/1 -> Add/1
  Constant1/1 -> Add/2
  Add/1 -> Sum/1
  Energy PI Control/1(pi_out) -> Mux4/1

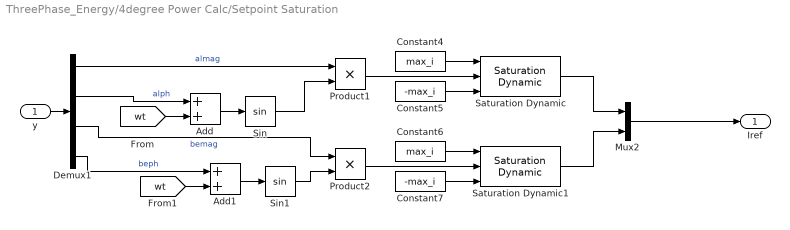
== system ThreePhase_Energy/4degree Power Calc/Setpoint Saturation ==
  y : Inport
  Add : Sum
  Add1 : Sum
  Constant4 : Constant  Value=max_i
  Constant5 : Constant  Value=-max_i
  Constant6 : Constant  Value=max_i
  Constant7 : Constant  Value=-max_i
  Demux1 : Demux
  Mux2 : Mux  Inputs=2
  Product1 : Product
  Product2 : Product
  Saturation Dynamic : simulink/Discontinuities/Saturation Dynamic  OutMin=[]  OutMax=[]  OutDataTypeStr=Inherit: Same as second input  OutDataType=fixdt(1, 16)  OutScaling=2^-10  DoSatur=off
  Saturation Dynamic1 : simulink/Discontinuities/Saturation Dynamic  OutMin=[]  OutMax=[]  OutDataTypeStr=Inherit: Same as second input  OutDataType=fixdt(1, 16)  OutScaling=2^-10  DoSatur=off
  Sin : Trigonometry
  Sin1 : Trigonometry
  Iref : Outport
  wires:
  Sin/1 -> Product1/2
  Constant4/1 -> Saturation Dynamic/1
  Saturation Dynamic/1 -> Mux2/1
  [wt] -> Add1/2
  Constant7/1 -> Saturation Dynamic1/3
  Demux1/2 -> Add/1  "alph"
  Add1/1 -> Sin1/1
  Saturation Dynamic1/1 -> Mux2/2
  Product1/1 -> Saturation Dynamic/2
  Constant6/1 -> Saturation Dynamic1/1
  Constant5/1 -> Saturation Dynamic/3
  Sin1/1 -> Product2/2
  Add/1 -> Sin/1
  Demux1/4 -> Add1/1  "beph"
  Demux1/3 -> Product2/1  "bemag"
  Product2/1 -> Saturation Dynamic1/2
  [wt] -> Add/2
  Demux1/1 -> Product1/1  "almag"
  y/1 -> Demux1/1
  Mux2/1 -> Iref/1

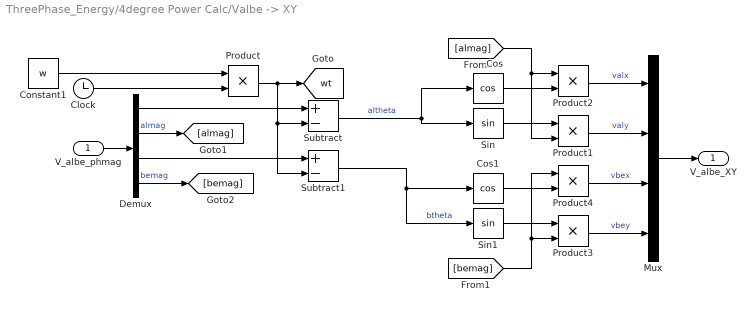
== system ThreePhase_Energy/4degree Power Calc/Valbe -> XY ==
  V_albe_phmag : Inport
  Clock : Clock
  Constant1 : Constant  Value=w
  Cos : Trigonometry  Operator=cos
  Cos1 : Trigonometry  Operator=cos
  Demux : Demux
  Mux : Mux
  Product{,1..4} (5 alike) : Product
  Sin : Trigonometry
  Sin1 : Trigonometry
  Subtract : Sum  Inputs=+-
  Subtract1 : Sum  Inputs=+-
  V_albe_XY : Outport
  tag scope: wt=global
  wires:
  Clock/1 -> Product/2
  Product/1 -> [wt], Subtract1/2, Subtract/2
  Subtract/1 -> Cos/1, Sin/1  "altheta"
  Demux/3 -> Subtract1/1
  Demux/1 -> Subtract/1
  Constant1/1 -> Product/1
  Demux/2 -> [almag]  "almag"
  Demux/4 -> [bemag]  "bemag"
  Subtract1/1 -> Cos1/1, Sin1/1  "btheta"
  V_albe_phmag/1 -> Demux/1
  Mux/1 -> V_albe_XY/1
  Sin/1 -> Product1/1
  Cos/1 -> Product2/2
  Cos1/1 -> Product4/2
  Sin1/1 -> Product3/1
  [almag] -> Product1/2, Product2/1
  [bemag] -> Product4/1, Product3/2
  Product1/1 -> Mux/2  "valy"
  Product2/1 -> Mux/1  "valx"
  Product4/1 -> Mux/3  "vbex"
  Product3/1 -> Mux/4  "vbey"

== system ThreePhase_Energy/4degree Power Calc/isetconv ==
  XY : Inport
  Mux4 : Mux
  almag : Fcn  Expr=sqrt(u(1)^2+u(2)^2)
  alph : Fcn  Expr=atan2(u(2),u(1))
  bemag : Fcn  Expr=sqrt(u(3)^2+u(4)^2)
  beph : Fcn  Expr=atan2(u(4),u(3))
  phmag : Outport
  wires:
  bemag/1 -> Mux4/3
  XY/1 -> alph/1, almag/1, bemag/1, beph/1
  almag/1 -> Mux4/1
  alph/1 -> Mux4/2
  beph/1 -> Mux4/4
  Mux4/1 -> phmag/1

== system ThreePhase_Energy/Current Control/PR ==
  ref : Inport
  meas : Inport  Port=2
  Add : Sum  Inputs=+++
  Gain2 : Gain  Gain=Kp
  Sum4 : Sum  Inputs=|-+
  ideal : TransferFcn  Numerator=[2*Ki 0]  Denominator=[1 0 w^2]
  nonideal1 : TransferFcn  Commented=on  Numerator=[2*Ki*wc 0]  Denominator=[1 2*wc w^2]
  out : Outport
  tag scope: e_ia=global
  wires:
  ref/1 -> Sum4/1
  meas/1 -> Sum4/2
  Add/1 -> out/1
  Gain2/1 -> Add/3
  ideal/1 -> Add/1
  Sum4/1 -> [e_ia], ideal/1, Gain2/1, nonideal1/1
  nonideal1/1 -> Add/2

== system ThreePhase_Energy/Current Control/PR1 ==
  ref : Inport
  meas : Inport  Port=2
  Add : Sum  Inputs=+++
  Gain2 : Gain  Gain=Kp
  Sum4 : Sum  Inputs=|-+
  ideal : TransferFcn  Numerator=[2*Ki 0]  Denominator=[1 0 w^2]
  nonideal1 : TransferFcn  Commented=on  Numerator=[2*Ki*wc 0]  Denominator=[1 2*wc w^2]
  out : Outport
  tag scope: e_ib=global
  wires:
  meas/1 -> Sum4/2
  ref/1 -> Sum4/1
  Sum4/1 -> nonideal1/1, Gain2/1, ideal/1, [e_ib]
  ideal/1 -> Add/1
  nonideal1/1 -> Add/2
  Add/1 -> out/1
  Gain2/1 -> Add/3

== system ThreePhase_Energy/Direct Current Ref Calc/PLL PI Control1 ==
  note: pi_out=(kp+ki/s)·pi_in
  pi_in : Inport
  Integrator : Integrator
  Sum : Sum
  ki : Gain  Gain=ki
  kp : Gain  Gain=kp
  pi_out : Outport
  wires:
  Sum/1 -> pi_out/1
  Integrator/1 -> Sum/2
  ki/1 -> Integrator/1
  kp/1 -> Sum/1
  pi_in/1 -> ki/1, kp/1

== system ThreePhase_Energy/Direct Current Ref Calc/PLL PI Control2 ==
  note: pi_out=(kp+ki/s)·pi_in
  pi_in : Inport
  Integrator : Integrator
  Sum : Sum
  ki : Gain  Gain=ki
  kp : Gain  Gain=kp
  pi_out : Outport
  wires:
  pi_in/1 -> kp/1, ki/1
  kp/1 -> Sum/1
  ki/1 -> Integrator/1
  Integrator/1 -> Sum/2
  Sum/1 -> pi_out/1

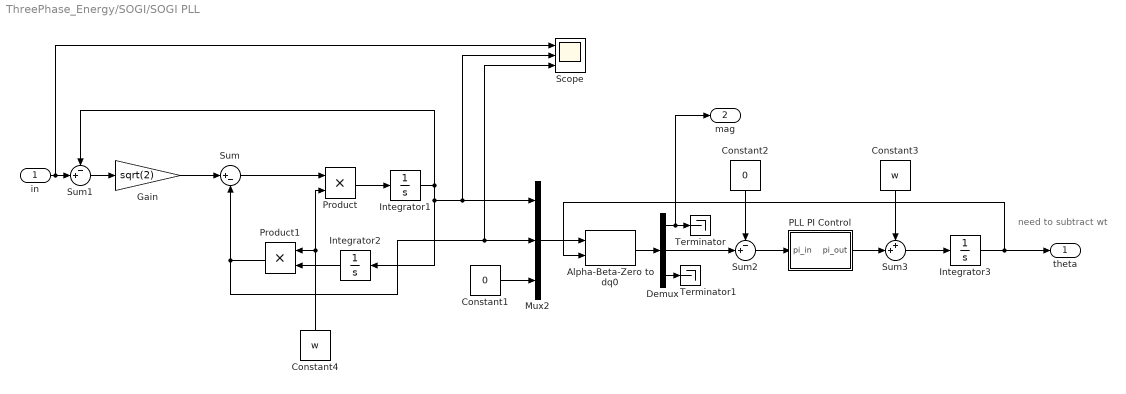
== system ThreePhase_Energy/SOGI/SOGI PLL ==
  note: need to subtract wt
  in : Inport
  Alpha-Beta-Zero to dq0 : spsAlphaBetaZerotodq0Lib/Alpha-Beta-Zero to dq0  Alignment=90 degrees behind phase A axis
  Constant1 : Constant  Value=0
  Constant2 : Constant  Value=0
  Constant3 : Constant  Value=w
  Constant4 : Constant  Value=w
  Demux : Demux  Outputs=3
  Gain : Gain  Gain=sqrt(2)
  Integrator1 : Integrator  InitialCondition=0.00001
  Integrator2 : Integrator  InitialCondition=0.00001
  Integrator3 : Integrator  InitialCondition=0.0031
  Mux2 : Mux  Inputs=3
  PLL PI Control : Subsystem
  Product : Product
  Product1 : Product
  Scope : Scope  NumInputPorts=3
  Sum : Sum  Inputs=|+-
  Sum1 : Sum  Inputs=-+|
  Sum2 : Sum  Inputs=-+|
  Sum3 : Sum  Inputs=++|
  Terminator : Terminator
  Terminator1 : Terminator
  theta : Outport
  mag : Outport  Port=2
  wires:
  Constant1/1 -> Mux2/3
  Alpha-Beta-Zero to dq0/1 -> Demux/1
  Demux/3 -> Terminator1/1
  Integrator3/1 -> theta/1, Alpha-Beta-Zero to dq0/2
  Gain/1 -> Sum/1
  Demux/2 -> Sum2/2
  Sum/1 -> Product/1
  Integrator1/1 -> Sum1/1, Scope/2, Mux2/1, Integrator2/1
  Product1/1 -> Scope/3, Mux2/2, Sum/2
  Demux/1 -> mag/1, Terminator/1
  Constant3/1 -> Sum3/1
  Sum1/1 -> Gain/1
  Constant2/1 -> Sum2/1
  Integrator2/1 -> Product1/2
  Sum2/1 -> PLL PI Control/1(pi_in)
  Mux2/1 -> Alpha-Beta-Zero to dq0/1
  Sum3/1 -> Integrator3/1
  Product/1 -> Integrator1/1
  PLL PI Control/1(pi_out) -> Sum3/2
  Constant4/1 -> Product/2, Product1/1
  in/1 -> Scope/1, Sum1/2

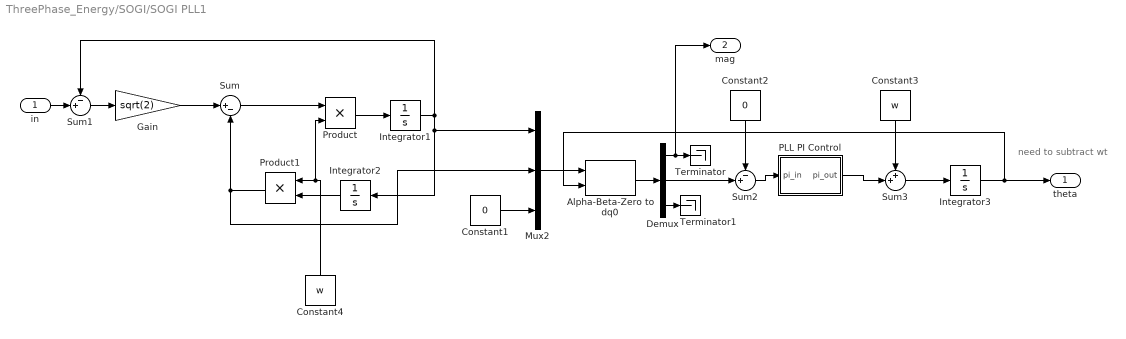
== system ThreePhase_Energy/SOGI/SOGI PLL1 ==
  note: need to subtract wt
  in : Inport
  Alpha-Beta-Zero to dq0 : spsAlphaBetaZerotodq0Lib/Alpha-Beta-Zero to dq0  Alignment=90 degrees behind phase A axis
  Constant1 : Constant  Value=0
  Constant2 : Constant  Value=0
  Constant3 : Constant  Value=w
  Constant4 : Constant  Value=w
  Demux : Demux  Outputs=3
  Gain : Gain  Gain=sqrt(2)
  Integrator1 : Integrator  InitialCondition=0.00001
  Integrator2 : Integrator  InitialCondition=0.00001
  Integrator3 : Integrator  InitialCondition=0.0031
  Mux2 : Mux  Inputs=3
  PLL PI Control : Subsystem
  Product : Product
  Product1 : Product
  Sum : Sum  Inputs=|+-
  Sum1 : Sum  Inputs=-+|
  Sum2 : Sum  Inputs=-+|
  Sum3 : Sum  Inputs=++|
  Terminator : Terminator
  Terminator1 : Terminator
  theta : Outport
  mag : Outport  Port=2
  wires:
  PLL PI Control/1(pi_out) -> Sum3/2
  Product/1 -> Integrator1/1
  Sum3/1 -> Integrator3/1
  Mux2/1 -> Alpha-Beta-Zero to dq0/1
  Sum2/1 -> PLL PI Control/1(pi_in)
  in/1 -> Sum1/2
  Integrator2/1 -> Product1/2
  Constant2/1 -> Sum2/1
  Sum1/1 -> Gain/1
  Constant3/1 -> Sum3/1
  Demux/1 -> Terminator/1, mag/1
  Product1/1 -> Sum/2, Mux2/2
  Integrator1/1 -> Integrator2/1, Mux2/1, Sum1/1
  Sum/1 -> Product/1
  Demux/2 -> Sum2/2
  Gain/1 -> Sum/1
  Integrator3/1 -> theta/1, Alpha-Beta-Zero to dq0/2
  Demux/3 -> Terminator1/1
  Alpha-Beta-Zero to dq0/1 -> Demux/1
  Constant1/1 -> Mux2/3
  Constant4/1 -> Product/2, Product1/1

== system ThreePhase_Energy/4degree Power Calc/Energy Control/Energy PI Control ==
  pi_in : Inport
  Integrator : Integrator
  Sum : Sum
  ki : Gain  Gain=eng_ki
  kp : Gain  Gain=eng_kp
  pi_out : Outport
  wires:
  pi_in/1 -> kp/1, ki/1
  kp/1 -> Sum/1
  ki/1 -> Integrator/1
  Integrator/1 -> Sum/2
  Sum/1 -> pi_out/1

== system ThreePhase_Energy/4degree Power Calc/Energy Control/Energy PI Control1 ==
  pi_in : Inport
  Integrator : Integrator
  Sum : Sum
  ki : Gain  Gain=eng_ki
  kp : Gain  Gain=eng_kp
  pi_out : Outport
  wires:
  Sum/1 -> pi_out/1
  Integrator/1 -> Sum/2
  ki/1 -> Integrator/1
  kp/1 -> Sum/1
  pi_in/1 -> ki/1, kp/1

== system ThreePhase_Energy/4degree Power Calc/Energy Control/Energy PI Control2 ==
  pi_in : Inport
  Integrator : Integrator
  Sum : Sum
  ki : Gain  Gain=eng_ki
  kp : Gain  Gain=eng_kp
  pi_out : Outport
  wires:
  pi_in/1 -> kp/1, ki/1
  kp/1 -> Sum/1
  ki/1 -> Integrator/1
  Integrator/1 -> Sum/2
  Sum/1 -> pi_out/1

== system ThreePhase_Energy/SOGI/SOGI PLL/PLL PI Control ==
  note: pi_out=(kp+ki/s)·pi_in
  pi_in : Inport
  Integrator : Integrator
  Sum : Sum
  ki : Gain  Gain=sogi_ki
  kp : Gain  Gain=sogi_kp
  pi_out : Outport
  wires:
  pi_in/1 -> kp/1, ki/1
  kp/1 -> Sum/1
  ki/1 -> Integrator/1
  Integrator/1 -> Sum/2
  Sum/1 -> pi_out/1

== system ThreePhase_Energy/SOGI/SOGI PLL1/PLL PI Control ==
  note: pi_out=(kp+ki/s)·pi_in
  pi_in : Inport
  Integrator : Integrator
  Sum : Sum
  ki : Gain  Gain=sogi_ki
  kp : Gain  Gain=sogi_kp
  pi_out : Outport
  wires:
  pi_in/1 -> kp/1, ki/1
  kp/1 -> Sum/1
  ki/1 -> Integrator/1
  Integrator/1 -> Sum/2
  Sum/1 -> pi_out/1
